simulink model "PID_ctrl_W6_03"  (R2021a)
settings: Solver=VariableStepAuto  StartTime=0.0  StopTime=300  RelTol=1e-3  EnableMultiTasking=on
undefined symbols (not defined in the file or in its folder): I, P
libraries: simulink_need_slupdate x1
settings Model: Creator=fo1521  LastModifiedBy=Ammar
settings SolverCC: ZeroCrossAlgorithm=Adaptive  AlgebraicLoopSolver=TrustRegion
settings DataIOCC: LimitDataPoints=on  SaveFormat=Array  SignalLoggingSaveFormat=ModelDataLogs  ReturnWorkspaceOutputs=off
settings OptimizationCC: ExpressionDepthLimit=2147483647  InitFltsAndDblsToZero=on  LifeSpan=inf
settings DebuggingCC: UnderspecifiedInitializationDetection=Classic  MergeDetectMultiDrivingBlocksExec=none  IgnoredZcDiagnostic=none  MultiTaskDSMMsg=warning  MultiTaskCondExecSysMsg=none  FcnCallInpInsideContextMsg=warning  StateNameClashWarn=warning  SFUnexpectedBacktrackingDiag=warning  SFNoUnconditionalDefaultTransitionDiag=warning  SFExecutionAtInitializationDiag=none  SFMachineParentedDataDiag=warning  ArithmeticOperatorsInVariantConditions=warning
settings HardwareCC: ProdBitPerPointer=32  ProdBitPerSizeT=32  ProdBitPerPtrDiffT=32  ProdLargestAtomicFloat=None  ProdIntDivRoundTo=Undefined  ProdEndianess=Unspecified  ProdWordSize=32  ProdHWDeviceType=32-bit Generic  TargetHWDeviceType=32-bit Generic
settings ModelReferenceCC: PropagateSignalLabelsOutOfModel=off
settings CodeAppCC: StateflowObjectComments=on
settings GRTTargetCC: TargetFcnLib=ansi_tfl_tmw.mat  TargetLangStandard=C89/C90 (ANSI)  CombineOutputUpdateFcns=off  GRTInterface=on
settings ConfigComp: CovMetricSettings=dw  CovSaveCumulativeToWorkspaceVar=on  CovSaveSingleToWorkspaceVar=on

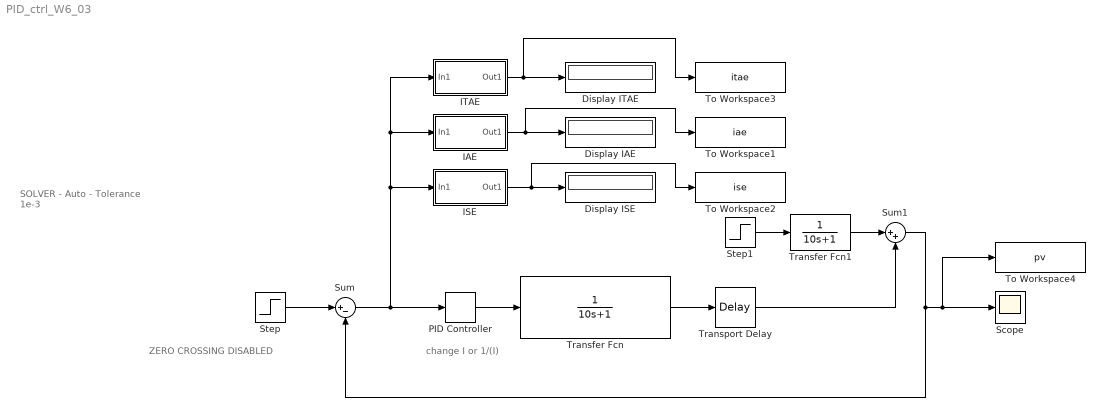
== system PID_ctrl_W6_03 ==
  note: change I or 1/(I)
  note: ZERO CROSSING DISABLED
  note: SOLVER
      |
      | - Auto
      | - Tolerance 1e-3
  Display IAE : Display
  Display ISE : Display
  Display ITAE : Display
  IAE : Subsystem
      mask help:
      | IAE performacne index
      |
      | output = int |input| dt
      mask Display:
      | disp('IAE')
      | port_label('input',1,'e')
      | port_label('output',1,'iae')
  ISE : Subsystem
      mask help:
      | ISE performance index
      |
      | output = int (input)^2 dt
      mask Display:
      | disp('ISE')
      | port_label('input',1,'e')
      | port_label('output',1,'ise')
  ITAE : Subsystem
      mask help:
      | ITAE performance index
      |
      | output = int t|input| dt
      mask Display:
      | disp('ITAE')
      | port_label('input',1,'e')
      | port_label('output',1,'itae')
  PID Controller : simulink_need_slupdate/PID Controller  P=P  I=1/(I)  D=0
  Scope : Scope
  Step : Step  After=4  SampleTime=1  ZeroCross=off
  Step1 : Step  SampleTime=0
  Sum : Sum  Inputs=|+-
  Sum1 : Sum  Inputs=|++
  To Workspace1 : ToWorkspace  VariableName=iae  SampleTime=1
  To Workspace2 : ToWorkspace  VariableName=ise  SampleTime=1
  To Workspace3 : ToWorkspace  VariableName=itae  SampleTime=1
  To Workspace4 : ToWorkspace  VariableName=pv  SampleTime=1
  Transfer Fcn : TransferFcn  Denominator=[10 1 ]
  Transfer Fcn1 : TransferFcn  Denominator=[10 1]
  Transport Delay : TransportDelay  DelayTime=2
  wires:
  PID Controller/1 -> Transfer Fcn/1
  Sum/1 -> PID Controller/1, ISE/1(In1), IAE/1(In1), ITAE/1(In1)
  Step/1 -> Sum/1
  IAE/1(Out1) -> To Workspace1/1, Display IAE/1
  Transfer Fcn/1 -> Transport Delay/1
  ISE/1(Out1) -> To Workspace2/1, Display ISE/1
  ITAE/1(Out1) -> To Workspace3/1, Display ITAE/1
  Step1/1 -> Transfer Fcn1/1
  Transport Delay/1 -> Sum1/2
  Sum1/1 -> To Workspace4/1, Scope/1, Sum/2
  Transfer Fcn1/1 -> Sum1/1

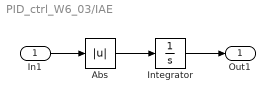
== system PID_ctrl_W6_03/IAE ==
  In1 : Inport
  Abs : Abs
  Integrator : Integrator
  Out1 : Outport
  wires:
  In1/1 -> Abs/1
  Integrator/1 -> Out1/1
  Abs/1 -> Integrator/1

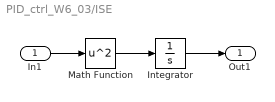
== system PID_ctrl_W6_03/ISE ==
  In1 : Inport
  Integrator : Integrator
  Math Function : Math  Operator=square  SignedPower=on  SaturateOnIntegerOverflow=on
  Out1 : Outport
  wires:
  Math Function/1 -> Integrator/1
  Integrator/1 -> Out1/1
  In1/1 -> Math Function/1

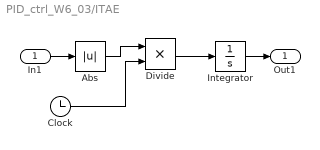
== system PID_ctrl_W6_03/ITAE ==
  In1 : Inport
  Abs : Abs
  Clock : Clock
  Divide : Product  Inputs=**
  Integrator : Integrator
  Out1 : Outport
  wires:
  Integrator/1 -> Out1/1
  In1/1 -> Abs/1
  Divide/1 -> Integrator/1
  Abs/1 -> Divide/1
  Clock/1 -> Divide/2
